simulink model "simple_quaternion_observer"  (R2024b)
settings: Solver=ode1  StartTime=0.0  StopTime=60  FixedStep=0.01  RelTol=1e-3
values from neighbouring files (symbols this model uses):
  F = 5    [assignment3.m]
undefined symbols (not defined in the file or in its folder): Light, MIL
libraries: aerolibutil x10, dspobslib x6, sharedutil x3, sharedtransform x3, matrix_library x2, simulink x1, robotcorelib x1, aerolibwind2 x1
settings Model: Creator=adan  LastModifiedBy=danyy
settings RTWCC: GPUComputeCapability=3.5

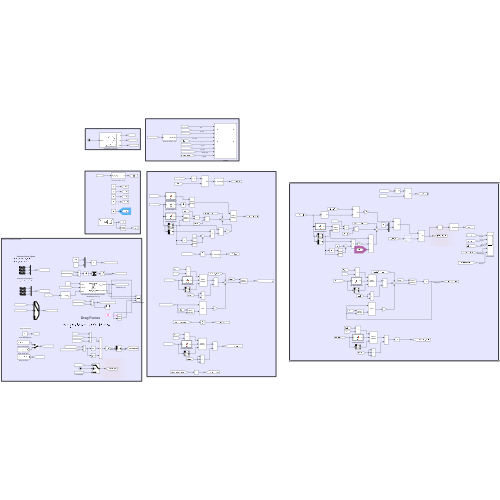
[thumbnail: Simulink's stored preview of the top-level diagram]
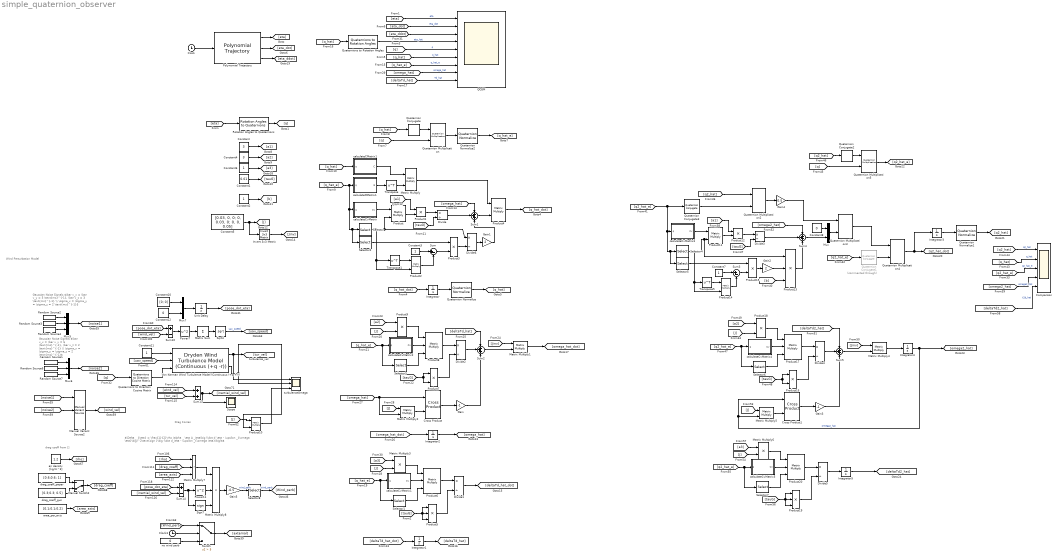
== system simple_quaternion_observer ==
  note: Gaussian Noise Signals
      | $\bar v_x = \bar v_y = 5 \text{ms}^{-1}, \bar v_z = 3 \text{ms}^{-1} \\ \sigma_x = \sigma_y = \sigma_z = 2 \text{ms}^{-1}$
  note: Drag Forces
  note: drag coeff from []
  note: Gaussian Noise Signals
      | $\bar v_x = \bar v_y = 6 \text{ms}^{-1}, \bar v_z = 2 \text{ms}^{-1} \\ \sigma_x = \sigma_y = \sigma_z = 2 \text{ms}^{-1}$
  note: $\Delta _ {\eta} = \frac{1}{2}\rho \alpha _ \eta A _\eta\big (\dot d_\eta - \upsilon _{\omega \eta}\big)^2\text{sign }\big (\dot d_\eta - \upsilon _{\omega \eta}\big)$$
  note: Wind Perturbation Model
  Clock : Clock
  Clock3 : Clock
  Comparison : Scope  NumInputPorts=5
  Constant : Constant  Value=3
  Constant1 : Constant  Value=0.01
  Constant10 : Constant  Value=[0; 0]
  Constant{2..3,6..7,11} (5 alike) : Constant
  Constant12 : Constant  Value=0
  Constant4 : Constant  Value=3
  Constant5 : Constant  Value=[0.03, 0, 0; 0, 0.03, 0; 0, 0, 0.05]
  Constant8 : Constant  Value=0
  Cross Product : matrix_library/Cross Product
  Cross Product1 : matrix_library/Cross Product
  Divide{,1..6} (7 alike) : Product  Inputs=*/
  Gain : Gain  Gain=-1
  Gain1 : Gain  Gain=2
  Gain2 : Gain  Gain=2
  Gain3 : Gain  Gain=-1
  Gain4 : Gain  Gain=0.5
  Gain5 : Gain  Gain=-0.5
  Integrator : Integrator  InitialCondition="[0.9995    0.0252    0.0146   -0.0144]'"
  Integrator{1..2,4..5} (4 alike) : Integrator  InitialCondition=[0; 0; 0]
  Integrator3 : Integrator  InitialCondition="[0.9995    0.0252    0.0146   -0.0144]'"
  Invert 3x3 Matrix : aerolibutil/Invert  3x3 Matrix
  Manual Variant Source2 : simulink/Signal Routing/Manual Variant Source  NumChoices=3  LabelModeActiveChoice=V_1
  Manual Switch2 : ManualSwitch  CurrentSetting=0
  Matrix Sum : Sum  Inputs=+
  Matrix Multiply{,1..2,4..5} (5 alike) : Product  Multiplication=Matrix(*)
  Matrix Multiply3 : Product
  Matrix Multiply6 : Product
  Matrix Multiply7 : Product  Inputs=3
  Matrix Multiply8 : Product  Inputs=3
  Mux : Mux  Inputs=2
  Mux5 : Mux  Inputs=3
  Mux6 : Mux  Inputs=3
  Mux7 : Mux  Inputs=2
  Polynomial Trajectory : robotcorelib/Polynomial Trajectory  WaypointSource=Internal  Waypoints=[0, 0, 0, 0, 0, 0; 0, 0, 0, 0.2, 0.2, 0; 0, 0.42, 0.78, 1.42, 3, 4]  TimePoints=[0, 12, 24, 36, 48, 60]  TimeInterval=[ 1, 4 ]  Method=Cubic Polynomial  ParameterSource=Internal  VelocityBoundaryCondition=zeros( 3, 6 )  AccelerationBoundaryCondition=zeros( 2, 5 )  SimulateUsing=Interpreted execution
  Power11 : Math  Operator=square
  Power7 : Math  Operator=square
  Product{,2,4,10..11,14} (6 alike) : Product  Multiplication=Matrix(*)
  Product{1,3,7,9,12,15..16,18} (8 alike) : Product
  Product13 : Product  Inputs=3
  Product{6,8,17,20} (4 alike) : Product  Inputs=3  Multiplication=Matrix(*)
  Product19 : Product  Inputs=3
  Product5 : Product  Inputs=3
  QOSM : Scope  NumInputPorts=9
  Quaternion Conjugate : aerolibutil/Quaternion Conjugate
  Quaternion Conjugate1 : aerolibutil/Quaternion Conjugate  Commented=through
  Quaternion Conjugate2 : aerolibutil/Quaternion Conjugate
  Quaternion Conjugate3 : aerolibutil/Quaternion Conjugate
  Quaternion Multiplication{,2..5} (5 alike) : aerolibutil/Quaternion Multiplication
  Quaternion Normalize : sharedutil/Quaternion Normalize  aMode=aMode
  Quaternion Normalize1 : sharedutil/Quaternion Normalize  aMode=aMode
  Quaternion Normalize2 : sharedutil/Quaternion Normalize  aMode=aMode
  Quaternions to Direction Cosine Matrix : sharedtransform/Quaternions to  Direction Cosine Matrix  aMode=aMode
      settings: LibrarySourceBlock=|
      | aerolibtransform2/Quaternions to
      | Direction Cosine Matrix
  Quaternions to Rotation Angles : sharedtransform/Quaternions to Rotation Angles  rotationOrder=XYZ  aMode=aMode
  Random Source2 : dspobslib/Random Source  SrcType=Gaussian  NormMethod=Ziggurat  CltLength=12  MinVal=0  MaxVal=1  MeanVal=5  VarVal=2  RepMode=Not repeatable  rawSeed=1  IsInherit=off  SampMode=Discrete  SampTime=0.01  SampFrame=1  DataType=Double  OutComplex=Real  OutputFrames=off
  Random Source3 : dspobslib/Random Source  SrcType=Gaussian  NormMethod=Ziggurat  CltLength=12  MinVal=0  MaxVal=1  MeanVal=5  VarVal=2  RepMode=Not repeatable  rawSeed=1  IsInherit=off  SampMode=Discrete  SampTime=0.01  SampFrame=1  DataType=Double  OutComplex=Real  OutputFrames=off
  Random Source4 : dspobslib/Random Source  SrcType=Gaussian  NormMethod=Ziggurat  CltLength=12  MinVal=0  MaxVal=1  MeanVal=3  VarVal=2  RepMode=Not repeatable  rawSeed=1  IsInherit=off  SampMode=Discrete  SampTime=0.01  SampFrame=1  DataType=Double  OutComplex=Real  OutputFrames=off
  Random Source5 : dspobslib/Random Source  SrcType=Gaussian  NormMethod=Ziggurat  CltLength=12  MinVal=0  MaxVal=1  MeanVal=6  VarVal=2  RepMode=Not repeatable  rawSeed=1  IsInherit=off  SampMode=Discrete  SampTime=1  SampFrame=1  DataType=Double  OutComplex=Real  OutputFrames=off
  Random Source6 : dspobslib/Random Source  SrcType=Gaussian  NormMethod=Ziggurat  CltLength=12  MinVal=0  MaxVal=1  MeanVal=6  VarVal=2  RepMode=Not repeatable  rawSeed=1  IsInherit=off  SampMode=Discrete  SampTime=1  SampFrame=1  DataType=Double  OutComplex=Real  OutputFrames=off
  Random Source7 : dspobslib/Random Source  SrcType=Gaussian  NormMethod=Ziggurat  CltLength=12  MinVal=0  MaxVal=1  MeanVal=2  VarVal=2  RepMode=Not repeatable  rawSeed=1  IsInherit=off  SampMode=Discrete  SampTime=1  SampFrame=1  DataType=Double  OutComplex=Real  OutputFrames=off
  Rotation Angles to Quaternions : sharedtransform/Rotation Angles to Quaternions  rotationOrder=XYZ  aMode=aMode
  Scope : Scope
  Selector{,1,3..4,6..7} (6 alike) : Selector  InputPortWidth=4  IndexOptions=Index vector (dialog)  Indices=[2:4]  OutputSizes=1
  Selector2 : Selector  InputPortWidth=4  IndexOptions=Index vector (dialog)  Indices=[1]  OutputSizes=1
  Selector5 : Selector  InputPortWidth=4  IndexOptions=Index vector (dialog)  Indices=[1]  OutputSizes=1
  Selector8 : Selector  InputPortWidth=3  IndexOptions=Index vector (dialog)  Indices=[3]  OutputSizes=1
  Sign7 : Signum
  Sqrt4 : Sqrt
  Sum : Sum  Inputs=|+-
  Sum{1..2,4..5} (4 alike) : Sum  Inputs=+++
  Sum10 : Sum  Inputs=+-
  Sum13 : Sum
  Sum14 : Sum  Inputs=+-
  Sum3 : Sum  Inputs=|+-
  Switch : Switch  Criteria=u2 > Threshold  Threshold=5  SaturateOnIntegerOverflow=off  InputSameDT=off
  Transpose : Math  Operator=transpose
  Transpose1 : Math  Operator=transpose
  Transpose5 : Math  Operator=transpose
  Unit Delay : UnitDelay  SampleTime=0.01  HasFrameUpgradeWarning=on
  Von Karman Wind Turbulence Model (Continuous (+q +r)) : aerolibwind2/Dryden Wind Turbulence Model  (Continuous (+q -r))  units=Metric (MKS)  spec=MIL-F-8785C  model=Continuous Von Karman (+q +r)  W20=15  Wdeg=0  TurbProb=10^-2 - Light  L_high=762  Wingspan=10  ts=0.1  Seed=[23341 23342 23343 23344]  T_on=on
      settings: LibrarySourceBlock=|
      | aerolibwind2/Von Karman Wind Turbulence Model
      | (Continuous (+q +r))
  air density [kg/m^3] : Constant  Value=1.2
  area_per_axis : Constant  Value=[0.1;0.1;0.2]
  calculateCMatrix1 : MATLAB Function  TreatAsAtomicUnit=on
  calculateCvMatrix : MATLAB Function  TreatAsAtomicUnit=on
  calculateCvMatrix1 : MATLAB Function  TreatAsAtomicUnit=on
  calculateCvMatrix2 : MATLAB Function  TreatAsAtomicUnit=on
  calculateCvMatrix3 : MATLAB Function  TreatAsAtomicUnit=on
  calculateCvMatrix4 : MATLAB Function  TreatAsAtomicUnit=on
  calculateCvMatrix5 : MATLAB Function  TreatAsAtomicUnit=on
  calculateGMatrix1 : MATLAB Function  TreatAsAtomicUnit=on
  drag_coeff_gus : Constant  Value=[0.3;0.3; 0.5]
  drag_coeff_paper : Constant  Value=[0.6;0.6; 1]
  no wind perb : Constant  Value=0
  turbulenceOmega : Scope  NumInputPorts=3
  wires:
  Clock/1 -> Polynomial Trajectory/1
  Polynomial Trajectory/3 -> [eta_ddot]
  Polynomial Trajectory/2 -> [eta_dot]
  Polynomial Trajectory/1 -> [eta]
  [eta] -> QOSM/1  "eta"
  [eta] -> Rotation Angles to Quaternions/1
  Rotation Angles to Quaternions/1 -> [q]
  [q] -> QOSM/5  "q"
  [q_hat_dot] -> Integrator/1
  Integrator/1 -> Quaternion Normalize/1
  Quaternion Normalize/1 -> [q_hat]
  [q_hat] -> QOSM/6  "q_hat"
  [eta_dot] -> QOSM/2  "eta_dot"
  Quaternion Conjugate/1 -> Quaternion Multiplication/1
  [q] -> Quaternion Multiplication/2
  [q_hat] -> Quaternion Conjugate/1
  Quaternion Multiplication/1 -> Quaternion Normalize2/1
  [q_hat_e] -> Selector2/1, Selector/1, calculateCvMatrix/1(q), calculateGMatrix1/1(q)
  [q_hat] -> calculateCMatrix1/1(q)
  calculateGMatrix1/1(G) -> Transpose/1
  Transpose/1 -> Matrix Multiply/2
  calculateCMatrix1/1(C) -> Matrix Multiply/1
  calculateCvMatrix/1(Cv) -> Product/1
  Selector/1 -> Divide6/1, Product/2, Product2/2, Transpose1/1
  Constant/1 -> [a1]
  Constant1/1 -> [tauG]
  Product/1 -> Product1/2
  [a1] -> Product1/1
  Product1/1 -> Divide/1
  [tauG] -> Divide/2
  Constant2/1 -> [b]
  Transpose1/1 -> Product2/1
  Constant3/1 -> Sum/1
  Product2/1 -> Sum/2
  Sum/1 -> Product3/2
  Selector2/1 -> Product3/1
  Divide/1 -> Sum1/2
  Sum1/1 -> Product4/2
  Matrix Multiply/1 -> Product4/1
  Product4/1 -> [q_hat_dot]
  [omega_hat] -> Sum1/1
  [q_hat_e] -> QOSM/7  "q_hat_e"
  [q_hat] -> Quaternions to Rotation Angles/1
  Quaternions to Rotation Angles/1 -> QOSM/4  "eta_hat"
  Constant5/1 -> Invert 3x3 Matrix/1, [J]
  Invert 3x3 Matrix/1 -> [Jinv]
  [deltaTd_hat_dot] -> Integrator1/1
  Integrator1/1 -> [deltaTd_hat]
  [deltaTd_hat] -> QOSM/9  "Td_hat"
  [tauG] -> Product5/3, Product5/1, Product5/2
  [q_hat_e] -> Selector1/1, calculateCvMatrix1/1(q)
  Selector1/1 -> Product6/3
  calculateCvMatrix1/1(Cv) -> Product6/2
  [J] -> Matrix Multiply3/2
  Product6/1 -> Divide1/1
  Product5/1 -> Divide1/2
  Divide1/1 -> [deltaTd_hat_dot]
  Product7/1 -> Divide2/2
  [q_hat_e] -> Selector3/1, calculateCvMatrix2/1(q)
  [tauG] -> Product7/2, Product7/1
  calculateCvMatrix2/1(Cv) -> Product8/2
  Selector3/1 -> Product8/3
  Product8/1 -> Divide2/1
  [J] -> Product9/2
  Product9/1 -> Product8/1
  [a2] -> Product9/1
  Integrator2/1 -> [omega_hat]
  Divide2/1 -> Sum2/2
  [deltaTd_hat] -> Sum2/1
  Sum2/1 -> Matrix Multiply1/2
  [Jinv] -> Matrix Multiply1/1
  Matrix Multiply1/1 -> [omega_hat_dot]
  [omega_hat_dot] -> Integrator2/1
  [omega_hat] -> Matrix Multiply2/2, Cross Product/1
  Matrix Multiply2/1 -> Cross Product/2
  [J] -> Matrix Multiply2/1
  Cross Product/1 -> Gain/1
  Gain/1 -> Sum2/3
  [omega_hat] -> QOSM/8  "omega_hat"
  Constant6/1 -> [a3]
  Constant4/1 -> [a2]
  [a3] -> Matrix Multiply3/1
  Matrix Multiply3/1 -> Product6/1
  [eta_ddot] -> QOSM/3
  Divide6/1 -> Gain1/1
  Product15/1 -> Gain2/1
  Product13/1 -> Sum4/3
  [a1] -> Product12/1
  Selector4/1 -> Product13/1, Product11/2, Product14/2, Transpose5/1
  [omega2_hat] -> Sum4/1
  Transpose5/1 -> Product14/1
  Product14/1 -> Sum3/2
  Divide3/1 -> Sum4/2
  [b] -> Product13/3
  [tauG] -> Divide3/2
  calculateCvMatrix3/1(Cv) -> Product11/1
  Constant7/1 -> Sum3/1
  Product12/1 -> Divide3/1
  Product11/1 -> Product12/2
  Sum3/1 -> Product15/2
  Selector5/1 -> Product15/1
  Gain2/1 -> Product13/2
  Sum4/1 -> Mux/2
  Constant8/1 -> Mux/1
  [q2_hat_e] -> Selector5/1, Selector4/1, calculateCvMatrix3/1(q), Quaternion Conjugate3/1
  [q2_hat] -> Quaternion Multiplication2/1
  Mux/1 -> Quaternion Multiplication3/2
  [q2_hat_e] -> Quaternion Conjugate1/1
  Quaternion Conjugate1/1 -> Quaternion Multiplication4/2
  Quaternion Multiplication3/1 -> Quaternion Multiplication4/1
  Quaternion Multiplication4/1 -> Integrator3/1, [q2_hat_dot]
  Integrator3/1 -> Quaternion Normalize1/1
  Quaternion Normalize1/1 -> [q2_hat]
  Quaternion Conjugate2/1 -> Quaternion Multiplication5/1
  [q2_hat] -> Quaternion Conjugate2/1
  Quaternion Multiplication5/1 -> [q2_hat_e]
  [q] -> Quaternion Multiplication5/2
  Quaternion Multiplication2/1 -> Gain4/1
  [q2_hat] -> Comparison/1  "q2_hat"
  [q_hat] -> Comparison/2  "q_hat"
  Quaternion Conjugate3/1 -> Quaternion Multiplication2/2
  [q2_hat_e] -> Comparison/3  "q2_hat_e"
  calculateCvMatrix4/1(Cv) -> Product17/2
  Divide4/1 -> Sum5/2
  [a2] -> Product18/1
  Cross Product1/1 -> Gain3/1
  Product17/1 -> Divide4/1
  Matrix Multiply5/1 -> Cross Product1/2
  Product18/1 -> Product17/1
  [tauG] -> Product16/2, Product16/1
  [q2_hat_e] -> Selector6/1, calculateCvMatrix4/1(q)
  Sum5/1 -> Matrix Multiply4/2
  Product16/1 -> Divide4/2
  Matrix Multiply4/1 -> Integrator4/1
  Integrator4/1 -> Cross Product1/1, Matrix Multiply5/2, [omega2_hat]  "omega2_hat"
  [J] -> Product18/2
  [Jinv] -> Matrix Multiply4/1
  Gain3/1 -> Sum5/3
  [J] -> Matrix Multiply5/1
  Selector6/1 -> Product17/3
  [omega2_hat] -> Comparison/4  "omega2_hat"
  Divide5/1 -> Integrator5/1
  Product19/1 -> Divide5/2
  Product20/1 -> Divide5/1
  [J] -> Matrix Multiply6/2
  Selector7/1 -> Product20/3
  [q2_hat_e] -> Selector7/1, calculateCvMatrix5/1(q)
  calculateCvMatrix5/1(Cv) -> Product20/2
  [tauG] -> Product19/3, Product19/1, Product19/2
  Matrix Multiply6/1 -> Product20/1
  [a3] -> Matrix Multiply6/1
  Integrator5/1 -> [deltaTd2_hat]
  [deltaTd2_hat] -> Sum5/1
  [deltaTd2_hat] -> Comparison/5  "t2d_hat"
  Gain4/1 -> Quaternion Multiplication3/1
  Quaternion Normalize2/1 -> [q_hat_e]
  Gain1/1 -> Sum1/3
  Product3/1 -> Divide6/2
  [tur_vel] -> Sum13/2
  drag_coeff_paper/1 -> Manual Switch2/1
  [pose_dot_eta] -> Sum14/1
  Power11/1 -> Matrix Multiply8/2
  Mux7/1 -> Unit Delay/1
  Sum10/1 -> Power7/1
  Sqrt4/1 -> [uav_speed]  "uav_speed"
  Manual Variant Source2/1 -> [wind_vel]
  Random Source7/1 -> Mux6/3
  Random Source6/1 -> Mux6/2
  Random Source5/1 -> Mux6/1
  Mux6/1 -> [noise2]
  Constant11/1 -> Von Karman Wind Turbulence Model (Continuous (+q +r))/1
  [wind_vel] -> Sum10/2
  Sum13/1 -> Scope/1, [inertial_wind_vel]
  [inertial_wind_vel] -> Sum14/2
  [uav_speed] -> Von Karman Wind Turbulence Model (Continuous (+q +r))/2
  Sum14/1 -> Sign7/1, Power11/1
  Power7/1 -> Matrix Sum/1
  Random Source3/1 -> Mux5/2
  Mux5/1 -> [noise1]
  Gain5/1 -> Selector8/1  "wind_perb"
  [rho] -> Matrix Multiply7/1
  drag_coeff_gus/1 -> Manual Switch2/2
  Switch/1 -> [external]
  air density [kg/m^3]/1 -> [rho]
  [noise2] -> Manual Variant Source2/2
  Matrix Sum/1 -> Sqrt4/1
  Clock3/1 -> Switch/2
  Von Karman Wind Turbulence Model (Continuous (+q +r))/1 -> turbulenceOmega/1, [tur_vel]
  [Wind_perb] -> Switch/1
  [pose_dot_eta] -> Sum10/1
  Matrix Multiply8/1 -> Gain5/1
  [area_axis] -> Matrix Multiply7/3
  Quaternions to Direction Cosine Matrix/1 -> Von Karman Wind Turbulence Model (Continuous (+q +r))/3
  Von Karman Wind Turbulence Model (Continuous (+q +r))/2 -> Product10/2, turbulenceOmega/2
  [noise1] -> Manual Variant Source2/1
  no wind perb/1 -> Switch/3
  Random Source2/1 -> Mux5/1
  Constant12/1 -> Mux7/2
  Random Source4/1 -> Mux5/3
  Selector8/1 -> [Wind_perb]  "wind_perb"
  Matrix Multiply7/1 -> Matrix Multiply8/1
  Constant10/1 -> Mux7/1
  area_per_axis/1 -> [area_axis]
  [drag_coeff] -> Matrix Multiply7/2
  Manual Switch2/1 -> [drag_coeff]
  Sign7/1 -> Matrix Multiply8/3
  [wind_vel] -> Sum13/1
  [q] -> Quaternions to Direction Cosine Matrix/1
  Unit Delay/1 -> [pose_dot_eta]
  [J] -> Product10/1
  Product10/1 -> turbulenceOmega/3

== matlab function simple_quaternion_observer/calculateGMatrix1 ==
  data: q input; G output
function G = fcn(q)

q0 = q(1);
q1 = q(2);
q2 = q(3);
q3 = q(4);

G = quat2rotm([q0 q1 q2 q3]);

== matlab function simple_quaternion_observer/calculateCvMatrix ==
  data: q input; Cv output
function Cv = fcn(q)

q0 = q(1);
q1 = q(2);
q2 = q(3);
q3 = q(4);

Cv = [q0, -q3, q2;
      q3, q0, -q1;
      -q2, q1, q0] * 0.5;

Cv = inv(Cv);

== matlab function simple_quaternion_observer/calculateCvMatrix1 ==
  data: q input; Cv output
function Cv = fcn(q)

q0 = q(1);
q1 = q(2);
q2 = q(3);
q3 = q(4);

Cv = [q0, -q3, q2;
      q3, q0, -q1;
      -q2, q1, q0] * 0.5;

Cv = pinv(Cv);

== matlab function simple_quaternion_observer/calculateCvMatrix2 ==
  data: q input; Cv output
function Cv = fcn(q)

q0 = q(1);
q1 = q(2);
q2 = q(3);
q3 = q(4);

Cv = [q0, -q3, q2;
      q3, q0, -q1;
      -q2, q1, q0] * 0.5;

Cv = pinv(Cv);

== matlab function simple_quaternion_observer/calculateCvMatrix4 ==
  data: q input; Cv output
function Cv = fcn(q)

q0 = q(1);
q1 = q(2);
q2 = q(3);
q3 = q(4);

Cv = [q0, -q3, q2;
      q3, q0, -q1;
      -q2, q1, q0] * 0.5;

Cv = pinv(Cv);

== matlab function simple_quaternion_observer/calculateCvMatrix5 ==
  data: q input; Cv output
function Cv = fcn(q)

q0 = q(1);
q1 = q(2);
q2 = q(3);
q3 = q(4);

Cv = [q0, -q3, q2;
      q3, q0, -q1;
      -q2, q1, q0] * 0.5;

Cv = pinv(Cv);

== matlab function simple_quaternion_observer/calculateCvMatrix3 ==
  data: q input; Cv output
function Cv = fcn(q)

q0 = q(1);
q1 = q(2);
q2 = q(3);
q3 = q(4);

Cv = [q0, -q3, q2;
      q3, q0, -q1;
      -q2, q1, q0] * 0.5;

Cv = pinv(Cv);

== matlab function simple_quaternion_observer/calculateCMatrix1 ==
  data: q input; C output
function C = fcn(q)

q0 = q(1);
q1 = q(2);
q2 = q(3);
q3 = q(4);

C = [-q1, -q2, -q3;
      q0, -q3, q2;
      q3, q0, -q1;
      -q2, q1, q0] * 0.5;
